simulink subsystem "ABB_irb120_qLC"  (R2023a)
settings: Solver=VariableStepAuto  StartTime=0.0  StopTime=10.0  RelTol=1e-3
model mask{baseRobot=baseRobot, q0_=q0_, Kq=Kq, Kw=Kw, Tsat=Tsat}
settings Model: DefaultTestHarness=Rob_qLC_Harness1  Creator=albher  LastModifiedBy=albher

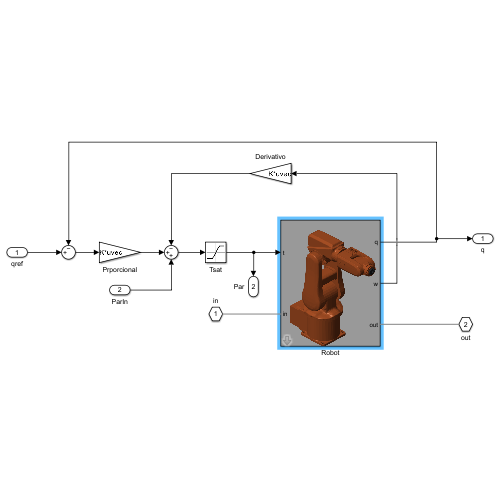
[thumbnail: Simulink's stored preview of the top-level diagram]
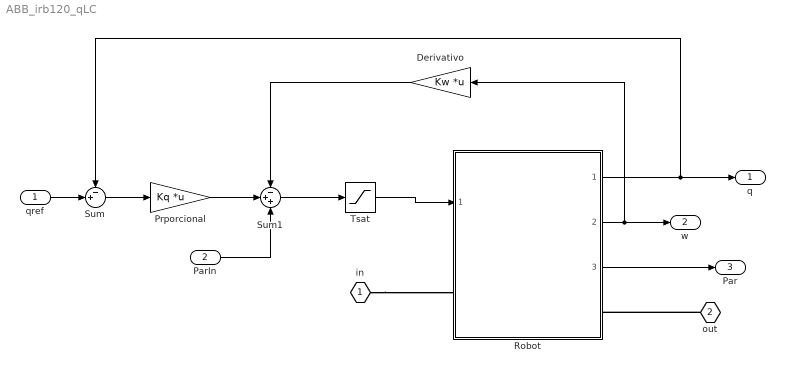
== system ABB_irb120_qLC ==
  qref : Inport  PortDimensions=6
  ParIn : Inport  Port=2
  Derivativo : Gain  Gain=Kw  Multiplication=Matrix(K*u) (u vector)
  Prporcional : Gain  Gain=Kq  Multiplication=Matrix(K*u) (u vector)
  Robot : Subsystem  ReferencedSubsystem=ABB_irb120_Din  baseRobot=baseRobot  q0_=q0_
  Sum : Sum  Inputs=-+|
  Sum1 : Sum  Inputs=-++
  Tsat : Saturate  UpperLimit=Tsat  LowerLimit=-Tsat
  in : PMIOPort  Side=Left
  out : PMIOPort  Port=2  Side=Right
  q : Outport
  w : Outport  Port=2
  Par : Outport  Port=3
  wires:
  Robot/1 -> Sum/1, q/1
  Derivativo/1 -> Sum1/1
  ParIn/1 -> Sum1/3
  qref/1 -> Sum/2
  Tsat/1 -> Robot/1
  Prporcional/1 -> Sum1/2
  Robot/2 -> Derivativo/1, w/1
  Robot/3 -> Par/1
  Sum1/1 -> Tsat/1
  Sum/1 -> Prporcional/1
  connections:
  in/RConn1 -- Robot/LConn1
  out/RConn1 -- Robot/RConn1
